simulink model "baseline_super_ground"  (R2021a)
settings: Solver=FixedStepAuto  StartTime=0.0  StopTime=50  FixedStep=framePeriod_s  RelTol=1e-3
undefined symbols (not defined in the file or in its folder): Aircraft, DiscIntNeverNeededParam, framePeriod_s
libraries: simulink x36
(part 1 of 2)
settings Model: Creator=brian  LastModifiedBy=Tuan Luong
settings SolverCC: AlgebraicLoopSolver=TrustRegion
settings OptimizationCC: DefaultParameterBehavior=Inlined  GainParamInheritBuiltInType=on  UseFloatMulNetSlope=on  DefaultUnderspecifiedDataType=single  InlineInvariantSignals=on  OptimizeBlockIOStorage=off  PassReuseOutputArgsAs=Individual arguments  ZeroExternalMemoryAtStartup=off  ZeroInternalMemoryAtStartup=off  NoFixptDivByZeroProtection=on  EfficientFloat2IntCast=on  LifeSpan=1  OptimizeBlockOrder=speed  DifferentSizesBufferReuse=on  EfficientTunableParamExpr=on
settings DebuggingCC: ParameterTunabilityLossMsg=error  SFMachineParentedDataDiag=warning
settings HardwareCC: ProdBitPerPointer=32  ProdBitPerSizeT=32  ProdBitPerPtrDiffT=32  ProdLargestAtomicInteger=Long  ProdLargestAtomicFloat=Double  ProdWordSize=32  ProdLongLongMode=on  ProdHWDeviceType=NXP->Cortex-M4
settings ModelReferenceCC: ModelReferenceNumInstancesAllowed=Single
settings SFSimCC: SimParseCustomCode=off  MATLABDynamicMemAlloc=off
settings RTWCC: SystemTargetFile=ert.tlc  GenCodeOnly=on  TemplateMakefile=ert_default_tmf  GenerateReport=on  RTWVerbose=off  Toolchain=Microsoft Visual C++ 2019 v16.0 | nmake (64-bit Windows)  BuildConfiguration=Faster Runs  IncludeHyperlinkInReport=on  TargetLang=C++  GenerateTraceInfo=on
settings CodeAppCC: ForceParamTrailComments=on  IgnoreCustomStorageClasses=off  OperatorAnnotations=on  SimulinkDataObjDesc=on  SFDataObjDesc=on  CustomSymbolStrGlobalVar=rt$N$M  CustomSymbolStrType=$N$M  CustomSymbolStrFcn=$N$M$F  CustomSymbolStrMacro=$N$M  InsertBlockDesc=on
settings ERTTargetCC: TargetLangStandard=C++03 (ISO)  IncludeMdlTerminateFcn=off  CombineSignalStateStructs=on  SuppressErrorStatus=on  SupportAbsoluteTime=off  CodeInterfacePackaging=C++ class  SupportComplex=off  ERTHeaderFileRootName=autocode$E  ERTSourceFileRootName=autocode$E  InlinedParameterPlacement=NonHierarchical  RootIOFormat=Structure reference  ERTCustomFileTemplate=example_file_process.tlc  ERTFilePackagingFormat=Compact  ArrayContainerType=std::array

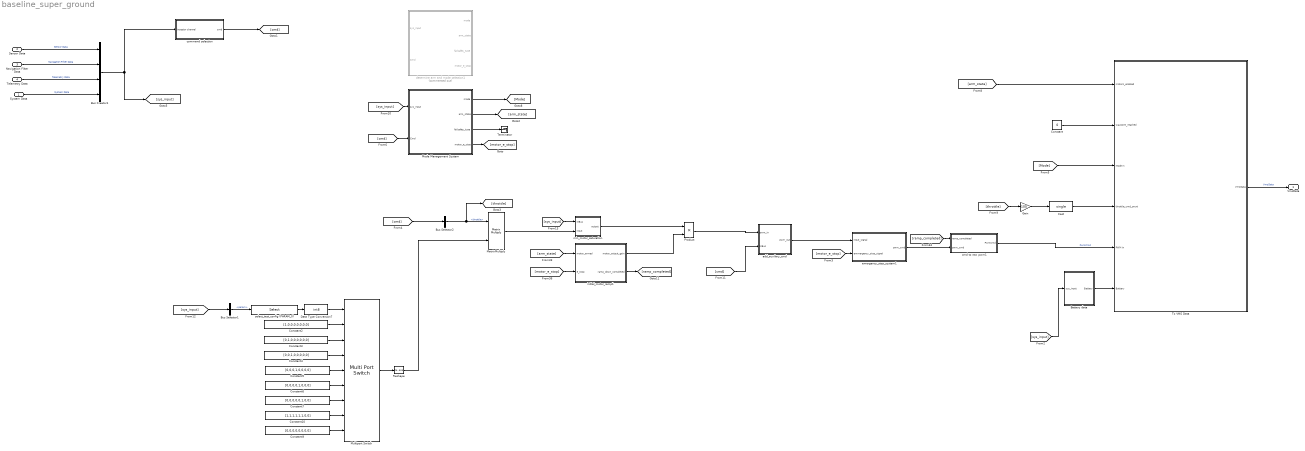
== system baseline_super_ground ==
  System Data : Inport  OutDataTypeStr=Bus: SysData  SampleTime=framePeriod_s  BusOutputAsStruct=on
  Sensor Data : Inport  Port=2  OutDataTypeStr=Bus: SensorData  SampleTime=framePeriod_s  BusOutputAsStruct=on
  Navigation Filter Data : Inport  Port=3  OutDataTypeStr=Bus: NavData  SampleTime=framePeriod_s  BusOutputAsStruct=on
  Telemetry Data : Inport  Port=4  OutDataTypeStr=Bus: TelemData  SampleTime=framePeriod_s  BusOutputAsStruct=on
  Battery data : Subsystem
  Bus Creator1 : BusCreator  Inputs=4
  Bus Selector1 : BusSelector  OutputSignals=Telemetry Data.param
  Bus Selector2 : BusSelector  OutputSignals=throttle
  Cast : DataTypeConversion  OutDataTypeStr=single
  Constant : Constant  Value=0  OutDataTypeStr=boolean
  Constant10 : Constant  Value=[1,1,1,1,1,1,0,0]  OutDataTypeStr=single
  Constant2 : Constant  Value=[1,0,0,0,0,0,0,0]  OutDataTypeStr=single
  Constant3 : Constant  Value=[0,1,0,0,0,0,0,0]  OutDataTypeStr=single
  Constant4 : Constant  Value=[0,0,1,0,0,0,0,0]  OutDataTypeStr=single
  Constant5 : Constant  Value=[0,0,0,1,0,0,0,0]  OutDataTypeStr=single
  Constant6 : Constant  Value=[0,0,0,0,1,0,0,0]  OutDataTypeStr=single
  Constant7 : Constant  Value=[0,0,0,0,0,1,0,0]  OutDataTypeStr=single
  Constant9 : Constant  Value=[0,0,0,0,0,0,0,0]  OutDataTypeStr=single
  Data Type Conversion7 : DataTypeConversion  OutDataTypeStr=int8
  Gain : Gain  Gain=100
  MatrixMultiply : Product  Multiplication=Matrix(*)
  Mode Management System : Subsystem
  Multiport Switch : MultiPortSwitch  DataPortOrder=Specify indices  Inputs=8  DataPortIndices={1,2,3,4,5,6,7}  DataPortForDefault=Additional data port
  Product : Product
  Reshape : Reshape  OutputDimensionality=Row vector (2-D)
  Terminator : Terminator
  To VMS Data : Subsystem
  add_auxilary_cmd : Subsystem
  cmd to raw pwm1 : Subsystem
  command selection : Subsystem
  determine arm and mode selection1 : Subsystem  Commented=on
  emergency_stop_system1 : Subsystem
  initial_motor_ramp1 : Subsystem
  min_motor_saturation : Subsystem
  select_test_config (PARAM_0) : Selector  IndexMode=Zero-based  IndexOptions=Index vector (dialog)  Indices=0  OutputSizes=1
  VmsData : Outport  OutDataTypeStr=Bus: VmsData  SampleTime=framePeriod_s  BusOutputAsStruct=on
  wires:
  Telemetry Data/1 -> Bus Creator1/3  "Telemetry Data"
  System Data/1 -> Bus Creator1/4  "System Data"
  Sensor Data/1 -> Bus Creator1/1  "Sensor Data"
  Navigation Filter Data/1 -> Bus Creator1/2  "Navigation Filter Data"
  To VMS Data/1(VmsData) -> VmsData/1  "VmsData"
  [Mode] -> To VMS Data/3(Mode in)
  Constant/1 -> To VMS Data/2(waypoint_reached)
  [arm_state] -> To VMS Data/1(motors_enabled)
  Cast/1 -> To VMS Data/4(throttle_cmd_prcnt)
  Battery data/1(Battery) -> To VMS Data/6(Battery)
  Bus Selector1/1 -> select_test_config (PARAM_0)/1  "<param>"
  select_test_config (PARAM_0)/1 -> Data Type Conversion7/1
  Data Type Conversion7/1 -> Multiport Switch/1
  [cmd] -> Bus Selector2/1
  Bus Selector2/1 -> [throttle], MatrixMultiply/1  "<throttle>"
  Multiport Switch/1 -> Reshape/1
  Reshape/1 -> MatrixMultiply/2
  [motor_e_stop] -> emergency_stop_system1/2(emmergency_stop_signal)
  initial_motor_ramp1/1(motor_output_gain) -> Product/2
  [sys_input] -> Battery data/1(sys_input)
  [throttle] -> Gain/1
  Gain/1 -> Cast/1
  Mode Management System/2(arm_state) -> [arm_state]
  command selection/1(cmd) -> [cmd]
  Mode Management System/3(failsafes_type) -> Terminator/1
  Mode Management System/1(mode) -> [Mode]
  Bus Creator1/1 -> command selection/1(inceptor channel), [sys_input]
  [cmd] -> Mode Management System/2(Cmd)
  [sys_input] -> Mode Management System/1(sys_input)
  Mode Management System/4(motor_e_stop) -> [motor_e_stop]
  Product/1 -> add_auxilary_cmd/1(pwm_in)
  add_auxilary_cmd/1(pwm_out) -> emergency_stop_system1/1(input_signal)
  [cmd] -> add_auxilary_cmd/2(InBus)
  Constant2/1 -> Multiport Switch/2
  Constant3/1 -> Multiport Switch/3
  Constant4/1 -> Multiport Switch/4
  Constant5/1 -> Multiport Switch/5
  Constant6/1 -> Multiport Switch/6
  Constant7/1 -> Multiport Switch/7
  Constant10/1 -> Multiport Switch/8
  Constant9/1 -> Multiport Switch/9
  [sys_input] -> Bus Selector1/1
  MatrixMultiply/1 -> min_motor_saturation/2(input)
  min_motor_saturation/1(output) -> Product/1
  [sys_input] -> min_motor_saturation/1(InBus)
  cmd to raw pwm1/1(PwmCmd) -> To VMS Data/5(PWM In)  "PwmCmd"
  emergency_stop_system1/1(pwm_cmd) -> cmd to raw pwm1/2(pwm_cmd)
  initial_motor_ramp1/2(ramp_down_completed) -> [ramp_completed]
  [arm_state] -> initial_motor_ramp1/1(motor_armed)
  [motor_e_stop] -> initial_motor_ramp1/2(e_stop)
  [ramp_completed] -> cmd to raw pwm1/1(ramp_completed)

== system baseline_super_ground/Battery data ==
  In Bus Element : Inport  PortName=sys_input  Element=Sensor Data.power_module.voltage_v
  In Bus Element1 : Inport  PortName=sys_input  Element=Sensor Data.power_module.current_v
  Bus Creator3 : BusCreator  Inputs=5  OutDataTypeStr=Bus: BatteryData  NonVirtualBus=on
  Discrete-Time Integrator : DiscreteIntegrator  IntegratorMethod=Integration: Trapezoidal  SampleTime=framePeriod_s  ICPrevOutput=DiscIntNeverNeededParam  ICPrevScaledInput=DiscIntNeverNeededParam
  Gain : Gain  Gain=Aircraft.Battery.voltage_gain
  Gain1 : Gain  Gain=Aircraft.Battery.current_to_voltage_gain_vpma
  remaining_prcnt : Constant  OutDataTypeStr=single
  remaining_time_s : Constant  OutDataTypeStr=single
  Battery : Outport
  wires:
  remaining_time_s/1 -> Bus Creator3/5  "remaining_time_s"
  Bus Creator3/1 -> Battery/1
  remaining_prcnt/1 -> Bus Creator3/4  "remaining_prcnt"
  In Bus Element1/1 -> Gain1/1
  Discrete-Time Integrator/1 -> Bus Creator3/3  "consumed_mah"
  In Bus Element/1 -> Gain/1
  Gain/1 -> Bus Creator3/1  "voltage_v"
  Gain1/1 -> Discrete-Time Integrator/1, Bus Creator3/2  "current_ma"

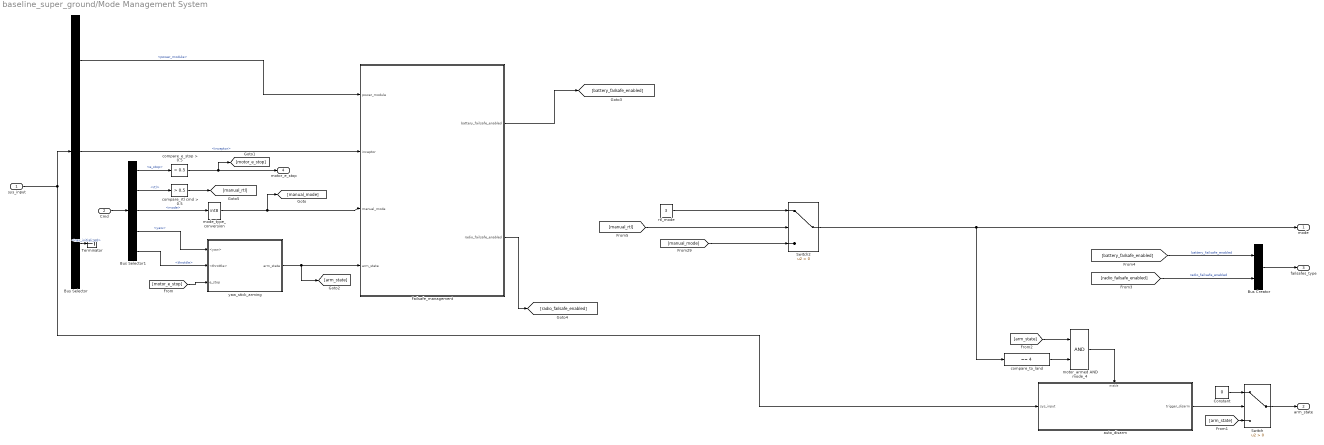
== system baseline_super_ground/Mode Management System ==
  sys_input : Inport
  Cmd : Inport  Port=2
  Bus Creator : BusCreator  Inputs=2
  Bus Selector : BusSelector  OutputSignals=Sensor Data.power_module,Sensor Data.inceptor,Navigation Filter Data.nav_initialized
  Bus Selector1 : BusSelector  OutputSignals=e_stop,rtl,mode,yaw,throttle
  Constant : Constant  Value=0  OutDataTypeStr=boolean
  Failsafe_management : Subsystem
  Switch : Switch  Criteria=u2 > Threshold
  Switch2 : Switch  Criteria=u2 > Threshold
  Terminator : Terminator
  auto_disarm : Subsystem
  compare_e_stop > 0.5 : simulink/Logic and Bit Operations/Compare To Constant  relop=>  const=0.5  OutDataTypeStr=boolean
  compare_rtl cmd > 0.5 : simulink/Logic and Bit Operations/Compare To Constant  relop=>  const=0.5  OutDataTypeStr=boolean
  compare_to_land : simulink/Logic and Bit Operations/Compare To Constant  relop===  const=4  OutDataTypeStr=boolean
  mode_type_conversion : DataTypeConversion  OutDataTypeStr=int8  RndMeth=Nearest
  motor_armed AND mode_4 : Logic  IconShape=distinctive  AllPortsSameDT=off  OutDataTypeStr=boolean
  rtl_mode : Constant  Value=3  OutDataTypeStr=int8
  yaw_stick_arming : Subsystem
  mode : Outport
  arm_state : Outport  Port=2
  failsafes_type : Outport  Port=3
  motor_e_stop : Outport  Port=4
  wires:
  mode_type_conversion/1 -> [manual_mode], Failsafe_management/3(manual_mode)
  rtl_mode/1 -> Switch2/1
  Failsafe_management/2(radio_failsafe_enabled) -> [radio_failsafe_enabled]
  [manual_mode] -> Switch2/3
  Failsafe_management/1(battery_failsafe_enabled) -> [battery_failsafe_enabled]
  Bus Selector/1 -> Failsafe_management/1(power_module)  "<power_module>"
  Bus Selector/2 -> Failsafe_management/2(inceptor)  "<inceptor>"
  sys_input/1 -> auto_disarm/1(sys_input), Bus Selector/1
  [arm_state] -> Switch/3
  auto_disarm/1(trigger_disarm) -> Switch/2
  Constant/1 -> Switch/1
  Switch/1 -> arm_state/1
  [arm_state] -> motor_armed AND mode_4/1
  compare_to_land/1 -> motor_armed AND mode_4/2
  Switch2/1 -> compare_to_land/1, mode/1
  motor_armed AND mode_4/1 -> auto_disarm/Enable
  [battery_failsafe_enabled] -> Bus Creator/1  "battery_failsafe_enabled"
  [radio_failsafe_enabled] -> Bus Creator/2  "radio_failsafe_enabled"
  Bus Creator/1 -> failsafes_type/1
  Cmd/1 -> Bus Selector1/1
  Bus Selector1/3 -> mode_type_conversion/1  "<mode>"
  Bus Selector1/2 -> compare_rtl cmd > 0.5/1  "<rtl>"
  compare_rtl cmd > 0.5/1 -> [manual_rtl]
  yaw_stick_arming/1(arm_state) -> Failsafe_management/4(arm_state), [arm_state]
  Bus Selector1/4 -> yaw_stick_arming/1(<yaw>)  "<yaw>"
  Bus Selector1/5 -> yaw_stick_arming/2(<throttle>)  "<throttle>"
  Bus Selector1/1 -> compare_e_stop > 0.5/1  "<e_stop>"
  compare_e_stop > 0.5/1 -> [motor_e_stop], motor_e_stop/1
  [manual_rtl] -> Switch2/2
  [motor_e_stop] -> yaw_stick_arming/3(e_stop)
  Bus Selector/3 -> Terminator/1  "<nav_initialized>"

== system baseline_super_ground/To VMS Data ==
  motors_enabled : Inport
  waypoint_reached : Inport  Port=2
  Mode in : Inport  Port=3
  throttle_cmd_prcnt : Inport  Port=4
  PWM In : Inport  Port=5
  Battery : Inport  Port=6
  Bus Creator : BusCreator  Inputs=9  OutDataTypeStr=Bus: VmsData  NonVirtualBus=on
  Bus Creator1 : BusCreator  Inputs=1  OutDataTypeStr=Bus: AnalogData
  Ground : Ground
  SBUS & AUX1 : Subsystem
  VmsData : Outport
  wires:
  waypoint_reached/1 -> Bus Creator/2  "waypoint_reached"
  Mode in/1 -> Bus Creator/3  "mode"
  motors_enabled/1 -> Bus Creator/1  "motors_enabled"
  Bus Creator/1 -> VmsData/1
  throttle_cmd_prcnt/1 -> Bus Creator/4  "throttle_cmd_prcnt"
  PWM In/1 -> Bus Creator/7  "pwm"
  SBUS & AUX1/1(aux) -> Bus Creator/5  "aux"
  SBUS & AUX1/2(sbus) -> Bus Creator/6  "SbusCmd"
  Battery/1 -> Bus Creator/9  "Battery"
  Bus Creator1/1 -> Bus Creator/8  "Analog"
  Ground/1 -> Bus Creator1/1  "val"

== system baseline_super_ground/add_auxilary_cmd ==
  pwm_in : Inport
  In Bus Element : Inport  Port=2  PortName=InBus  Element=engine
  In Bus Element1 : Inport  Port=2  PortName=InBus  Element=relay
  Demux : Demux  Outputs=8
  Mux : Mux  Inputs=8
  Sum : Sum  Inputs=|++
  Sum1 : Sum  Inputs=|++
  pwm_out : Outport
  wires:
  Demux/1 -> Mux/1  "motor1"
  Demux/2 -> Mux/2  "motor2"
  Demux/3 -> Mux/3  "motor3"
  Demux/6 -> Mux/6  "motor6"
  Demux/4 -> Mux/4  "motor4"
  Demux/5 -> Mux/5  "motor5"
  Mux/1 -> pwm_out/1
  pwm_in/1 -> Demux/1
  Demux/7 -> Sum/1
  Sum/1 -> Mux/7  "relay"
  Demux/8 -> Sum1/1
  Sum1/1 -> Mux/8  "engine"
  In Bus Element1/1 -> Sum/2
  In Bus Element/1 -> Sum1/2

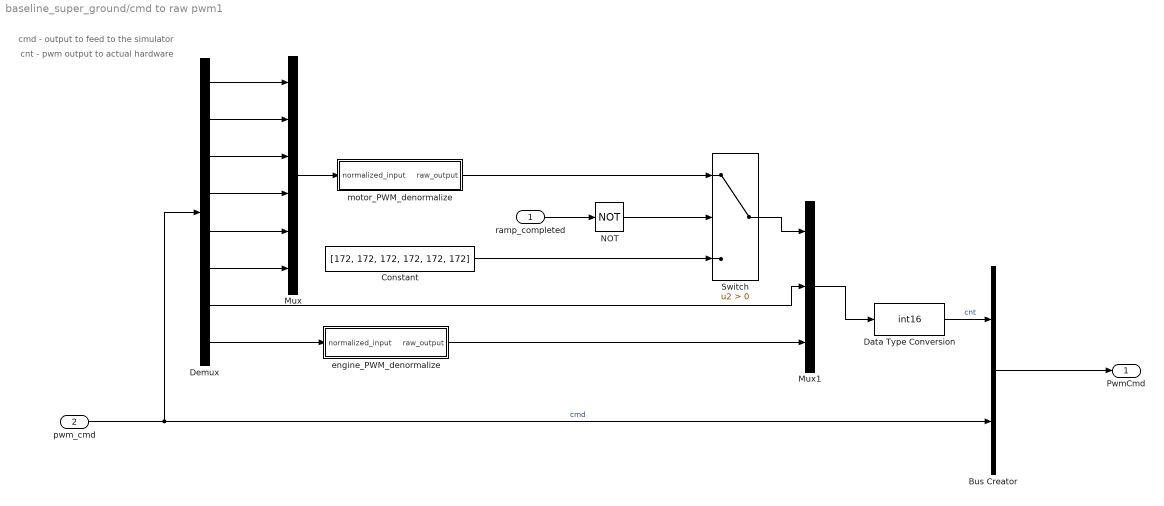
== system baseline_super_ground/cmd to raw pwm1 ==
  note: cnt - pwm output to actual hardware
  note: cmd - output to feed to the simulator
  ramp_completed : Inport
  pwm_cmd : Inport  Port=2
  Bus Creator : BusCreator  Inputs=2  OutDataTypeStr=Bus: PwmCmd  NonVirtualBus=on
      settings: InheritFromInputs=off
  Constant : Constant  Value=[172, 172, 172, 172, 172, 172]
  Data Type Conversion : DataTypeConversion  OutDataTypeStr=int16
  Demux : Demux  Outputs=8
  Mux : Mux  Inputs=6
  Mux1 : Mux  Inputs=3
  NOT : Logic  Operator=NOT  IconShape=distinctive  AllPortsSameDT=off  OutDataTypeStr=boolean
  Switch : Switch  Criteria=u2 > Threshold
  engine_PWM_denormalize : Subsystem
  motor_PWM_denormalize : Subsystem
  PwmCmd : Outport
  wires:
  Mux1/1 -> Data Type Conversion/1
  engine_PWM_denormalize/1(raw_output) -> Mux1/3
  Demux/7 -> Mux1/2
  Switch/1 -> Mux1/1
  Demux/8 -> engine_PWM_denormalize/1(normalized_input)
  motor_PWM_denormalize/1(raw_output) -> Switch/1
  Mux/1 -> motor_PWM_denormalize/1(normalized_input)
  Demux/6 -> Mux/6
  Demux/5 -> Mux/5
  Demux/4 -> Mux/4
  Demux/3 -> Mux/3
  Demux/2 -> Mux/2
  Demux/1 -> Mux/1
  Constant/1 -> Switch/3
  Data Type Conversion/1 -> Bus Creator/1  "cnt"
  pwm_cmd/1 -> Bus Creator/2, Demux/1  "cmd"
  Bus Creator/1 -> PwmCmd/1
  ramp_completed/1 -> NOT/1
  NOT/1 -> Switch/2

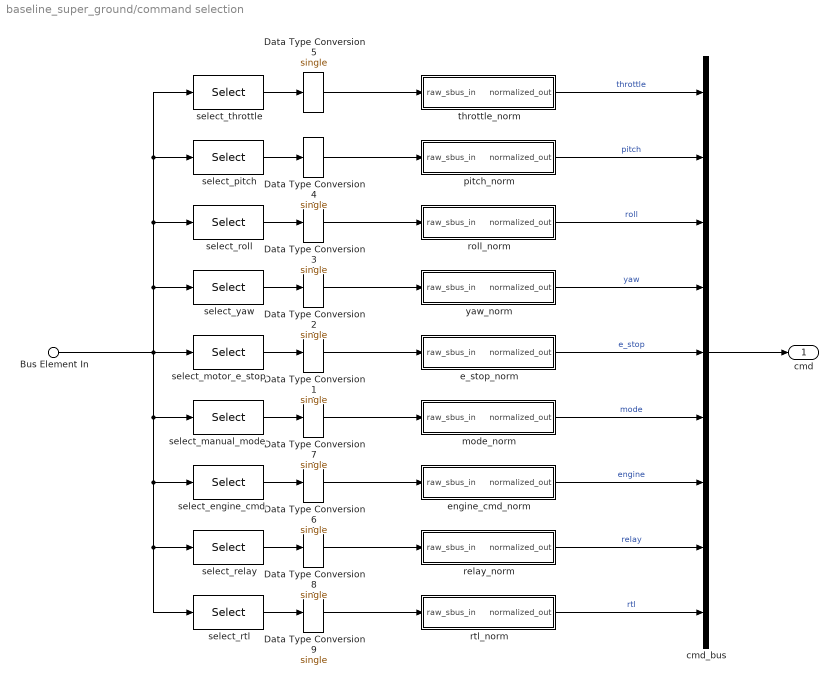
== system baseline_super_ground/command selection ==
  Bus Element In : Inport  PortName=inceptor channel  Element=Sensor Data.inceptor.ch
  Data Type Conversion{1..9} (9 alike) : DataTypeConversion  OutDataTypeStr=single
  cmd_bus : BusCreator  Inputs=9
  e_stop_norm : Subsystem
  engine_cmd_norm : Subsystem
  mode_norm : Subsystem
  pitch_norm : Subsystem
  relay_norm : Subsystem
  roll_norm : Subsystem
  rtl_norm : Subsystem
  select_engine_cmd : Selector  IndexOptions=Index vector (dialog)  Indices=Aircraft.Inceptor.engine_cmd  OutputSizes=1
  select_manual_mode : Selector  IndexOptions=Index vector (dialog)  Indices=Aircraft.Inceptor.mode0  OutputSizes=1
  select_motor_e_stop : Selector  IndexOptions=Index vector (dialog)  Indices=Aircraft.Inceptor.throttle_e_stop  OutputSizes=1
  select_pitch : Selector  IndexOptions=Index vector (dialog)  Indices=Aircraft.Inceptor.pitch  OutputSizes=1
  select_relay : Selector  IndexOptions=Index vector (dialog)  Indices=Aircraft.Inceptor.relay  OutputSizes=1
  select_roll : Selector  IndexOptions=Index vector (dialog)  Indices=Aircraft.Inceptor.roll  OutputSizes=1
  select_rtl : Selector  IndexOptions=Index vector (dialog)  Indices=Aircraft.Inceptor.rtl  OutputSizes=1
  select_throttle : Selector  IndexOptions=Index vector (dialog)  Indices=Aircraft.Inceptor.throttle  OutputSizes=1
  select_yaw : Selector  IndexOptions=Index vector (dialog)  Indices=Aircraft.Inceptor.yaw  OutputSizes=1
  throttle_norm : Subsystem
  yaw_norm : Subsystem
  cmd : Outport
  wires:
  select_pitch/1 -> Data Type Conversion4/1
  select_yaw/1 -> Data Type Conversion2/1
  Data Type Conversion2/1 -> yaw_norm/1(raw_sbus_in)
  select_throttle/1 -> Data Type Conversion5/1
  Data Type Conversion4/1 -> pitch_norm/1(raw_sbus_in)
  cmd_bus/1 -> cmd/1
  Data Type Conversion3/1 -> roll_norm/1(raw_sbus_in)
  Data Type Conversion5/1 -> throttle_norm/1(raw_sbus_in)
  select_roll/1 -> Data Type Conversion3/1
  Bus Element In/1 -> select_relay/1, select_rtl/1, select_engine_cmd/1, select_manual_mode/1, select_throttle/1, select_pitch/1, select_roll/1, select_yaw/1, select_motor_e_stop/1
  Data Type Conversion1/1 -> e_stop_norm/1(raw_sbus_in)
  select_motor_e_stop/1 -> Data Type Conversion1/1
  select_engine_cmd/1 -> Data Type Conversion6/1
  Data Type Conversion6/1 -> engine_cmd_norm/1(raw_sbus_in)
  Data Type Conversion7/1 -> mode_norm/1(raw_sbus_in)
  select_manual_mode/1 -> Data Type Conversion7/1
  select_relay/1 -> Data Type Conversion8/1
  Data Type Conversion8/1 -> relay_norm/1(raw_sbus_in)
  select_rtl/1 -> Data Type Conversion9/1
  Data Type Conversion9/1 -> rtl_norm/1(raw_sbus_in)
  throttle_norm/1(normalized_out) -> cmd_bus/1  "throttle"
  pitch_norm/1(normalized_out) -> cmd_bus/2  "pitch"
  roll_norm/1(normalized_out) -> cmd_bus/3  "roll"
  yaw_norm/1(normalized_out) -> cmd_bus/4  "yaw"
  e_stop_norm/1(normalized_out) -> cmd_bus/5  "e_stop"
  mode_norm/1(normalized_out) -> cmd_bus/6  "mode"
  engine_cmd_norm/1(normalized_out) -> cmd_bus/7  "engine"
  relay_norm/1(normalized_out) -> cmd_bus/8  "relay"
  rtl_norm/1(normalized_out) -> cmd_bus/9  "rtl"

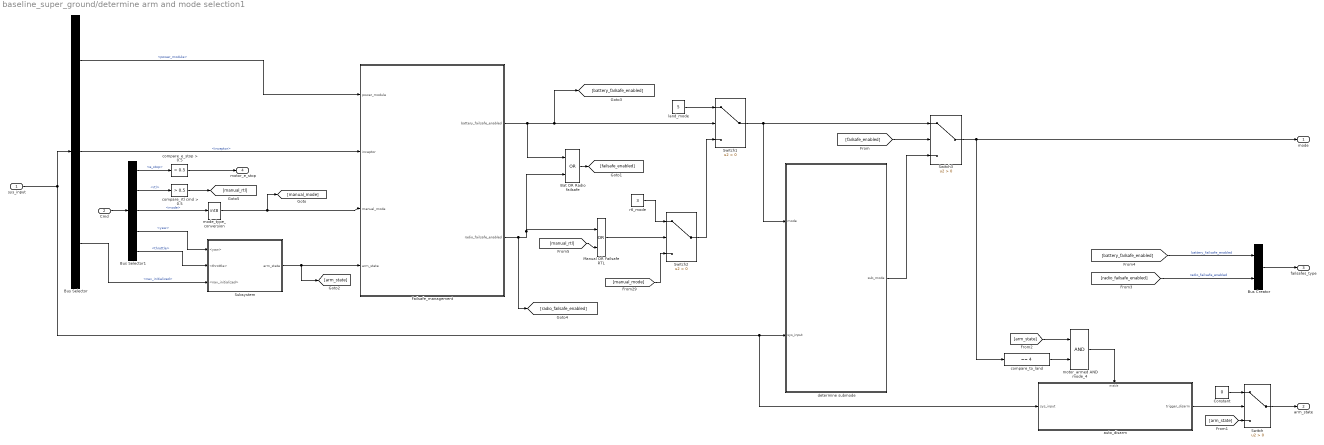
== system baseline_super_ground/determine arm and mode selection1 ==
  sys_input : Inport
  Cmd : Inport  Port=2
  Bat OR Radio failsafe : Logic  Operator=OR  IconShape=distinctive  AllPortsSameDT=off  OutDataTypeStr=boolean
  Bus Creator : BusCreator  Inputs=2
  Bus Selector : BusSelector  OutputSignals=Sensor Data.power_module,Sensor Data.inceptor,Navigation Filter Data.nav_initialized
  Bus Selector1 : BusSelector  OutputSignals=e_stop,rtl,mode,yaw,throttle
  Constant : Constant  Value=0  OutDataTypeStr=boolean
  Failsafe_management : Subsystem
  Manual OR Failsafe RTL : Logic  Operator=OR  IconShape=distinctive  AllPortsSameDT=off  OutDataTypeStr=boolean
  Subsystem : Subsystem
  Switch{,1..3} (4 alike) : Switch  Criteria=u2 > Threshold
  auto_disarm : Subsystem
  compare_e_stop > 0.5 : simulink/Logic and Bit Operations/Compare To Constant  relop=>  const=0.5  OutDataTypeStr=boolean
  compare_rtl cmd > 0.5 : simulink/Logic and Bit Operations/Compare To Constant  relop=>  const=0.5  OutDataTypeStr=boolean
  compare_to_land : simulink/Logic and Bit Operations/Compare To Constant  relop===  const=4  OutDataTypeStr=boolean
  determine submode : Subsystem
  land_mode : Constant  Value=5  OutDataTypeStr=int8
  mode_type_conversion : DataTypeConversion  OutDataTypeStr=int8  RndMeth=Nearest
  motor_armed AND mode_4 : Logic  IconShape=distinctive  AllPortsSameDT=off  OutDataTypeStr=boolean
  rtl_mode : Constant  Value=3  OutDataTypeStr=int8
  mode : Outport
  arm_state : Outport  Port=2
  failsafes_type : Outport  Port=3
  motor_e_stop : Outport  Port=4
  wires:
  mode_type_conversion/1 -> [manual_mode], Failsafe_management/3(manual_mode)
  rtl_mode/1 -> Switch2/1
  Failsafe_management/2(radio_failsafe_enabled) -> Bat OR Radio failsafe/2, Manual OR Failsafe RTL/1, [radio_failsafe_enabled]
  [manual_mode] -> Switch2/3
  land_mode/1 -> Switch1/1
  Failsafe_management/1(battery_failsafe_enabled) -> [battery_failsafe_enabled], Switch1/2, Bat OR Radio failsafe/1
  Bus Selector/3 -> Subsystem/3(<nav_initialized>)  "<nav_initialized>"
  Bus Selector/1 -> Failsafe_management/1(power_module)  "<power_module>"
  Bus Selector/2 -> Failsafe_management/2(inceptor)  "<inceptor>"
  Switch2/1 -> Switch1/3
  Bat OR Radio failsafe/1 -> [failsafe_enabled]
  sys_input/1 -> determine submode/2(sys_input), auto_disarm/1(sys_input), Bus Selector/1
  [failsafe_enabled] -> Switch3/2
  Switch1/1 -> Switch3/1, determine submode/1(mode)
  determine submode/1(sub_mode) -> Switch3/3
  [arm_state] -> Switch/3
  auto_disarm/1(trigger_disarm) -> Switch/2
  Constant/1 -> Switch/1
  Switch/1 -> arm_state/1
  [arm_state] -> motor_armed AND mode_4/1
  compare_to_land/1 -> motor_armed AND mode_4/2
  Switch3/1 -> compare_to_land/1, mode/1
  motor_armed AND mode_4/1 -> auto_disarm/Enable
  [battery_failsafe_enabled] -> Bus Creator/1  "battery_failsafe_enabled"
  [radio_failsafe_enabled] -> Bus Creator/2  "radio_failsafe_enabled"
  Bus Creator/1 -> failsafes_type/1
  Cmd/1 -> Bus Selector1/1
  Bus Selector1/3 -> mode_type_conversion/1  "<mode>"
  Manual OR Failsafe RTL/1 -> Switch2/2
  [manual_rtl] -> Manual OR Failsafe RTL/2
  Bus Selector1/2 -> compare_rtl cmd > 0.5/1  "<rtl>"
  compare_rtl cmd > 0.5/1 -> [manual_rtl]
  Subsystem/1(arm_state) -> Failsafe_management/4(arm_state), [arm_state]
  Bus Selector1/4 -> Subsystem/1(<yaw>)  "<yaw>"
  Bus Selector1/5 -> Subsystem/2(<throttle>)  "<throttle>"
  Bus Selector1/1 -> compare_e_stop > 0.5/1  "<e_stop>"
  compare_e_stop > 0.5/1 -> motor_e_stop/1

== system baseline_super_ground/emergency_stop_system1 ==
  input_signal : Inport
  emmergency_stop_signal : Inport  Port=2
  Constant : Constant  Value=[0,0,0,0,0,0,0,0]  OutDataTypeStr=single
  emergency_switch : Switch  Criteria=u2 > Threshold  Threshold=0.5
  pwm_cmd : Outport
  wires:
  emergency_switch/1 -> pwm_cmd/1
  emmergency_stop_signal/1 -> emergency_switch/2
  Constant/1 -> emergency_switch/1
  input_signal/1 -> emergency_switch/3

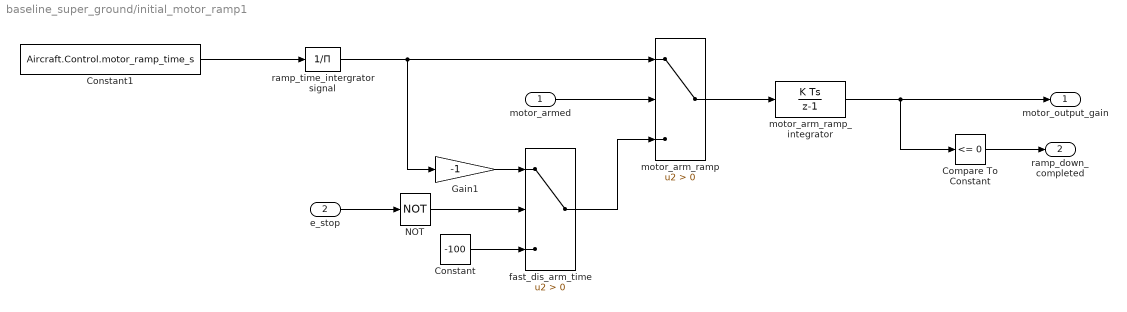
== system baseline_super_ground/initial_motor_ramp1 ==
  motor_armed : Inport
  e_stop : Inport  Port=2
  Compare To Constant : simulink/Logic and Bit Operations/Compare To Constant  relop=<=  const=0  OutDataTypeStr=boolean
  Constant : Constant  Value=-100
  Constant1 : Constant  Value=Aircraft.Control.motor_ramp_time_s  OutDataTypeStr=single
  Gain1 : Gain  Gain=-1
  NOT : Logic  Operator=NOT  IconShape=distinctive  AllPortsSameDT=off  OutDataTypeStr=boolean
  fast_dis_arm_time : Switch  Criteria=u2 > Threshold
  motor_arm_ramp : Switch  Criteria=u2 > Threshold
  motor_arm_ramp_integrator : DiscreteIntegrator  SampleTime=framePeriod_s  LimitOutput=on  UpperSaturationLimit=1  LowerSaturationLimit=0  ICPrevOutput=DiscIntNeverNeededParam  ICPrevScaledInput=DiscIntNeverNeededParam
  ramp_time_intergrator signal : Product  Inputs=/
  motor_output_gain : Outport
  ramp_down_completed : Outport  Port=2
  wires:
  Constant1/1 -> ramp_time_intergrator signal/1
  motor_arm_ramp/1 -> motor_arm_ramp_integrator/1
  ramp_time_intergrator signal/1 -> Gain1/1, motor_arm_ramp/1
  motor_arm_ramp_integrator/1 -> Compare To Constant/1, motor_output_gain/1
  motor_armed/1 -> motor_arm_ramp/2
  e_stop/1 -> NOT/1
  NOT/1 -> fast_dis_arm_time/2
  fast_dis_arm_time/1 -> motor_arm_ramp/3
  Gain1/1 -> fast_dis_arm_time/1
  Constant/1 -> fast_dis_arm_time/3
  Compare To Constant/1 -> ramp_down_completed/1

== system baseline_super_ground/min_motor_saturation ==
  In Bus Element : Inport  PortName=InBus  Element=Telemetry Data.param
  input : Inport  Port=2
  Constant : Constant
  Saturation Dynamic : simulink/Discontinuities/Saturation Dynamic  OutMin=[]  OutMax=[]  OutDataTypeStr=Inherit: Same as second input  OutDataType=fixdt(1, 16)  OutScaling=2^-10  DoSatur=off
  "min_motor_throttle (PARAM_1) " : Selector  IndexMode=Zero-based  IndexOptions=Index vector (dialog)  Indices=1  OutputSizes=1
  output : Outport
  wires:
  Constant/1 -> Saturation Dynamic/1
  input/1 -> Saturation Dynamic/2
  "min_motor_throttle (PARAM_1) "/1 -> Saturation Dynamic/3
  Saturation Dynamic/1 -> output/1
  In Bus Element/1 -> "min_motor_throttle (PARAM_1) "/1

== system baseline_super_ground/Mode Management System/Failsafe_management ==
  note: - radio failsafe
      | - battery failsafe
  Bus Element In : Inport  PortName=power_module  Element=voltage_v
  Bus Element In1 : Inport  Port=2  PortName=inceptor  Element=failsafe
  manual_mode : Inport  Port=3
  arm_state : Inport  Port=4
  Battery failsafe : Subsystem
  Radio failsafe : Subsystem
  battery_failsafe_enabled : Outport
  radio_failsafe_enabled : Outport  Port=2
  wires:
  Radio failsafe/1(radio_failsafe_enabled) -> radio_failsafe_enabled/1
  Battery failsafe/1(battery_failsafe_enabled) -> battery_failsafe_enabled/1
  manual_mode/1 -> [manual_mode], Radio failsafe/2(manual_mode)
  arm_state/1 -> Radio failsafe/3(arm_state), Battery failsafe/1(arm_state)
  [manual_mode] -> Battery failsafe/3(manual_mode)
  Bus Element In/1 -> Battery failsafe/2(voltage_v)
  Bus Element In1/1 -> Radio failsafe/1(failsafe)

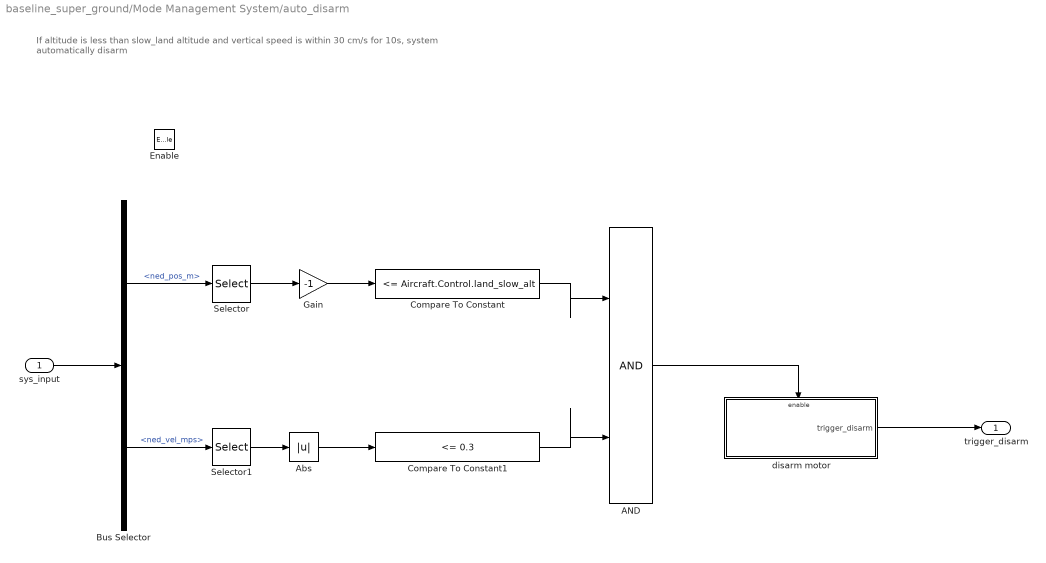
== system baseline_super_ground/Mode Management System/auto_disarm ==
  note: If altitude is less than slow_land altitude and vertical speed is within 30 cm/s for 10s, system automatically disarm
  sys_input : Inport
  Enable : EnablePort
  AND : Logic  IconShape=distinctive  AllPortsSameDT=off  OutDataTypeStr=boolean
  Abs : Abs
  Bus Selector : BusSelector  OutputSignals=Navigation Filter Data.ned_pos_m,Navigation Filter Data.ned_vel_mps
  Compare To Constant : simulink/Logic and Bit Operations/Compare To Constant  relop=<=  const=Aircraft.Control.land_slow_alt  OutDataTypeStr=boolean
  Compare To Constant1 : simulink/Logic and Bit Operations/Compare To Constant  relop=<=  const=0.3  OutDataTypeStr=boolean
  Gain : Gain  Gain=-1
  Selector : Selector  InputPortWidth=3  IndexOptions=Index vector (dialog)  Indices=3  OutputSizes=1
  Selector1 : Selector  InputPortWidth=3  IndexOptions=Index vector (dialog)  Indices=3  OutputSizes=1
  disarm motor : Subsystem
  trigger_disarm : Outport
  wires:
  sys_input/1 -> Bus Selector/1
  Bus Selector/1 -> Selector/1  "<ned_pos_m>"
  Bus Selector/2 -> Selector1/1  "<ned_vel_mps>"
  Selector/1 -> Gain/1
  Gain/1 -> Compare To Constant/1
  Selector1/1 -> Abs/1
  Abs/1 -> Compare To Constant1/1
  Compare To Constant/1 -> AND/1
  Compare To Constant1/1 -> AND/2
  AND/1 -> disarm motor/Enable
  disarm motor/1(trigger_disarm) -> trigger_disarm/1

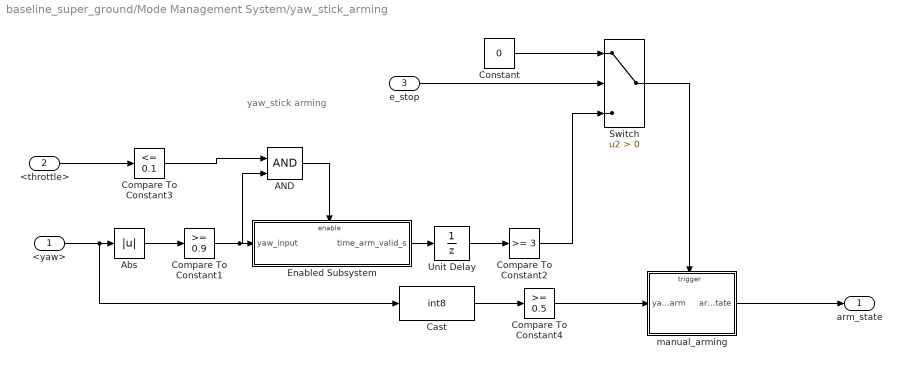
== system baseline_super_ground/Mode Management System/yaw_stick_arming ==
  note: yaw_stick arming
  <yaw> : Inport
  <throttle> : Inport  Port=2
  e_stop : Inport  Port=3
  AND : Logic  IconShape=distinctive  AllPortsSameDT=off  OutDataTypeStr=boolean
  Abs : Abs
  Cast : DataTypeConversion  OutDataTypeStr=int8
  Compare To Constant1 : simulink/Logic and Bit Operations/Compare To Constant  relop=>=  const=0.9  OutDataTypeStr=boolean
  Compare To Constant2 : simulink/Logic and Bit Operations/Compare To Constant  relop=>=  const=3  OutDataTypeStr=boolean
  Compare To Constant3 : simulink/Logic and Bit Operations/Compare To Constant  relop=<=  const=0.1  OutDataTypeStr=boolean
  Compare To Constant4 : simulink/Logic and Bit Operations/Compare To Constant  relop=>=  const=0.5  OutDataTypeStr=boolean
  Constant : Constant  Value=0  OutDataTypeStr=boolean  LockScale=on
  Enabled Subsystem : Subsystem  TreatAsAtomicUnit=on
  Switch : Switch  Criteria=u2 > Threshold
  Unit Delay : UnitDelay  SampleTime=-1  HasFrameUpgradeWarning=on
  manual_arming : Subsystem
  arm_state : Outport
  wires:
  Unit Delay/1 -> Compare To Constant2/1
  Abs/1 -> Compare To Constant1/1
  Enabled Subsystem/1(time_arm_valid_s) -> Unit Delay/1
  Compare To Constant1/1 -> AND/2, Enabled Subsystem/1(yaw_input)
  Compare To Constant4/1 -> manual_arming/1(yaw_arm)
  AND/1 -> Enabled Subsystem/Enable
  Cast/1 -> Compare To Constant4/1
  manual_arming/1(arm_state) -> arm_state/1
  <throttle>/1 -> Compare To Constant3/1
  <yaw>/1 -> Cast/1, Abs/1
  Switch/1 -> manual_arming/Trigger
  e_stop/1 -> Switch/2
  Constant/1 -> Switch/1
  Compare To Constant2/1 -> Switch/3
  Compare To Constant3/1 -> AND/1

== system baseline_super_ground/To VMS Data/SBUS & AUX1 ==
  Bus Creator : BusCreator  Inputs=4  OutDataTypeStr=Bus: SbusCmd  NonVirtualBus=on
  Constant : Constant  Value=0  OutDataTypeStr=boolean
  Constant1 : Constant  Value=0  OutDataTypeStr=boolean
  Data Type Conversion1 : DataTypeConversion  OutDataTypeStr=single
  Ground : Ground
  Ground1 : Ground
  Ground2 : Ground
  aux : Outport
  sbus : Outport  Port=2  SampleTime=framePeriod_s
  wires:
  Ground/1 -> Data Type Conversion1/1
  Data Type Conversion1/1 -> aux/1
  Bus Creator/1 -> sbus/1
  Constant/1 -> Bus Creator/1  "ch17"
  Constant1/1 -> Bus Creator/2  "ch18"
  Ground1/1 -> Bus Creator/3  "cnt"
  Ground2/1 -> Bus Creator/4  "cmd"

== system baseline_super_ground/cmd to raw pwm1/engine_PWM_denormalize ==
  normalized_input : Inport
  Constant : Constant  Value=0  OutDataTypeStr=single
  Constant1 : Constant  Value=900  OutDataTypeStr=single
  Constant2 : Constant  Value=2100  OutDataTypeStr=single
  Constant3 : Constant  OutDataTypeStr=single
  remap : MATLAB Function  TreatAsAtomicUnit=on
  raw_output : Outport
  wires:
  Constant2/1 -> remap/5(out_max)
  Constant1/1 -> remap/4(out_min)
  Constant3/1 -> remap/3(in_max)
  Constant/1 -> remap/2(in_min)
  remap/1(raw_out) -> raw_output/1
  normalized_input/1 -> remap/1(norm_in)

== system baseline_super_ground/cmd to raw pwm1/motor_PWM_denormalize ==
  normalized_input : Inport
  Constant : Constant  Value=0  OutDataTypeStr=single
  Constant1 : Constant  Value=1100  OutDataTypeStr=single
  Constant2 : Constant  Value=1900  OutDataTypeStr=single
  Constant3 : Constant  OutDataTypeStr=single
  remap : MATLAB Function  TreatAsAtomicUnit=on
  raw_output : Outport
  wires:
  Constant2/1 -> remap/5(out_max)
  Constant1/1 -> remap/4(out_min)
  Constant3/1 -> remap/3(in_max)
  Constant/1 -> remap/2(in_min)
  remap/1(raw_out) -> raw_output/1
  normalized_input/1 -> remap/1(norm_in)

== system baseline_super_ground/command selection/e_stop_norm ==
  raw_sbus_in : Inport
  Constant : Constant  Value=172  OutDataTypeStr=single
  Constant1 : Constant  Value=0  OutDataTypeStr=single
  Constant2 : Constant  OutDataTypeStr=single
  Constant3 : Constant  Value=1811  OutDataTypeStr=single
  remap : MATLAB Function  TreatAsAtomicUnit=on
  normalized_out : Outport
  wires:
  Constant2/1 -> remap/5(out_max)
  Constant1/1 -> remap/4(out_min)
  Constant3/1 -> remap/3(in_max)
  Constant/1 -> remap/2(in_min)
  remap/1(norm_out) -> normalized_out/1
  raw_sbus_in/1 -> remap/1(raw_in)

== system baseline_super_ground/command selection/engine_cmd_norm ==
  raw_sbus_in : Inport
  Constant : Constant  Value=172  OutDataTypeStr=single
  Constant1 : Constant  Value=0  OutDataTypeStr=single
  Constant2 : Constant  OutDataTypeStr=single
  Constant3 : Constant  Value=1811  OutDataTypeStr=single
  remap : MATLAB Function  TreatAsAtomicUnit=on
  normalized_out : Outport
  wires:
  Constant2/1 -> remap/5(out_max)
  Constant1/1 -> remap/4(out_min)
  Constant3/1 -> remap/3(in_max)
  Constant/1 -> remap/2(in_min)
  remap/1(norm_out) -> normalized_out/1
  raw_sbus_in/1 -> remap/1(raw_in)

== system baseline_super_ground/command selection/mode_norm ==
  raw_sbus_in : Inport
  Constant : Constant  Value=172  OutDataTypeStr=single
  Constant1 : Constant  Value=0  OutDataTypeStr=single
  Constant2 : Constant  Value=2  OutDataTypeStr=single
  Constant3 : Constant  Value=1811  OutDataTypeStr=single
  remap : MATLAB Function  TreatAsAtomicUnit=on
  normalized_out : Outport
  wires:
  raw_sbus_in/1 -> remap/1(raw_in)
  remap/1(norm_out) -> normalized_out/1
  Constant/1 -> remap/2(in_min)
  Constant3/1 -> remap/3(in_max)
  Constant1/1 -> remap/4(out_min)
  Constant2/1 -> remap/5(out_max)

== system baseline_super_ground/command selection/pitch_norm ==
  raw_sbus_in : Inport
  Constant : Constant  Value=172  OutDataTypeStr=single
  Constant1 : Constant  Value=-1  OutDataTypeStr=single
  Constant2 : Constant  OutDataTypeStr=single
  Constant3 : Constant  Value=1811  OutDataTypeStr=single
  remap : MATLAB Function  TreatAsAtomicUnit=on
  normalized_out : Outport
  wires:
  raw_sbus_in/1 -> remap/1(raw_in)
  remap/1(norm_out) -> normalized_out/1
  Constant/1 -> remap/2(in_min)
  Constant3/1 -> remap/3(in_max)
  Constant1/1 -> remap/4(out_min)
  Constant2/1 -> remap/5(out_max)

== system baseline_super_ground/command selection/relay_norm ==
  raw_sbus_in : Inport
  Constant : Constant  Value=172  OutDataTypeStr=single
  Constant1 : Constant  Value=0  OutDataTypeStr=single
  Constant2 : Constant  OutDataTypeStr=single
  Constant3 : Constant  Value=1811  OutDataTypeStr=single
  remap : MATLAB Function  TreatAsAtomicUnit=on
  normalized_out : Outport
  wires:
  raw_sbus_in/1 -> remap/1(raw_in)
  remap/1(norm_out) -> normalized_out/1
  Constant/1 -> remap/2(in_min)
  Constant3/1 -> remap/3(in_max)
  Constant1/1 -> remap/4(out_min)
  Constant2/1 -> remap/5(out_max)

== system baseline_super_ground/command selection/roll_norm ==
  raw_sbus_in : Inport
  Constant : Constant  Value=172  OutDataTypeStr=single
  Constant1 : Constant  Value=-1  OutDataTypeStr=single
  Constant2 : Constant  OutDataTypeStr=single
  Constant3 : Constant  Value=1811  OutDataTypeStr=single
  remap : MATLAB Function  TreatAsAtomicUnit=on
  normalized_out : Outport
  wires:
  Constant2/1 -> remap/5(out_max)
  Constant1/1 -> remap/4(out_min)
  Constant3/1 -> remap/3(in_max)
  Constant/1 -> remap/2(in_min)
  remap/1(norm_out) -> normalized_out/1
  raw_sbus_in/1 -> remap/1(raw_in)

== system baseline_super_ground/command selection/rtl_norm ==
  raw_sbus_in : Inport
  Constant : Constant  Value=172  OutDataTypeStr=single
  Constant1 : Constant  Value=0  OutDataTypeStr=single
  Constant2 : Constant  OutDataTypeStr=single
  Constant3 : Constant  Value=1811  OutDataTypeStr=single
  remap : MATLAB Function  TreatAsAtomicUnit=on
  normalized_out : Outport
  wires:
  Constant2/1 -> remap/5(out_max)
  Constant1/1 -> remap/4(out_min)
  Constant3/1 -> remap/3(in_max)
  Constant/1 -> remap/2(in_min)
  remap/1(norm_out) -> normalized_out/1
  raw_sbus_in/1 -> remap/1(raw_in)

== system baseline_super_ground/command selection/throttle_norm ==
  raw_sbus_in : Inport
  Constant : Constant  Value=172  OutDataTypeStr=single
  Constant1 : Constant  Value=0  OutDataTypeStr=single
  Constant2 : Constant  OutDataTypeStr=single
  Constant3 : Constant  Value=1811  OutDataTypeStr=single
  remap : MATLAB Function  TreatAsAtomicUnit=on
  normalized_out : Outport
  wires:
  raw_sbus_in/1 -> remap/1(raw_in)
  remap/1(norm_out) -> normalized_out/1
  Constant/1 -> remap/2(in_min)
  Constant3/1 -> remap/3(in_max)
  Constant1/1 -> remap/4(out_min)
  Constant2/1 -> remap/5(out_max)

== system baseline_super_ground/command selection/yaw_norm ==
  raw_sbus_in : Inport
  Constant : Constant  Value=172  OutDataTypeStr=single
  Constant1 : Constant  Value=-1  OutDataTypeStr=single
  Constant2 : Constant  OutDataTypeStr=single
  Constant3 : Constant  Value=1811  OutDataTypeStr=single
  remap : MATLAB Function  TreatAsAtomicUnit=on
  normalized_out : Outport
  wires:
  raw_sbus_in/1 -> remap/1(raw_in)
  remap/1(norm_out) -> normalized_out/1
  Constant/1 -> remap/2(in_min)
  Constant3/1 -> remap/3(in_max)
  Constant1/1 -> remap/4(out_min)
  Constant2/1 -> remap/5(out_max)

== system baseline_super_ground/determine arm and mode selection1/Failsafe_management ==
  note: - radio failsafe
      | - battery failsafe
  Bus Element In : Inport  PortName=power_module  Element=voltage_v
  Bus Element In1 : Inport  Port=2  PortName=inceptor  Element=failsafe
  manual_mode : Inport  Port=3
  arm_state : Inport  Port=4
  Battery failsafe : Subsystem
  Radio failsafe : Subsystem
  battery_failsafe_enabled : Outport
  radio_failsafe_enabled : Outport  Port=2
  wires:
  Radio failsafe/1(radio_failsafe_enabled) -> radio_failsafe_enabled/1
  Battery failsafe/1(battery_failsafe_enabled) -> battery_failsafe_enabled/1
  manual_mode/1 -> [manual_mode], Radio failsafe/2(manual_mode)
  arm_state/1 -> Radio failsafe/3(arm_state), Battery failsafe/1(arm_state)
  [manual_mode] -> Battery failsafe/3(manual_mode)
  Bus Element In/1 -> Battery failsafe/2(voltage_v)
  Bus Element In1/1 -> Radio failsafe/1(failsafe)

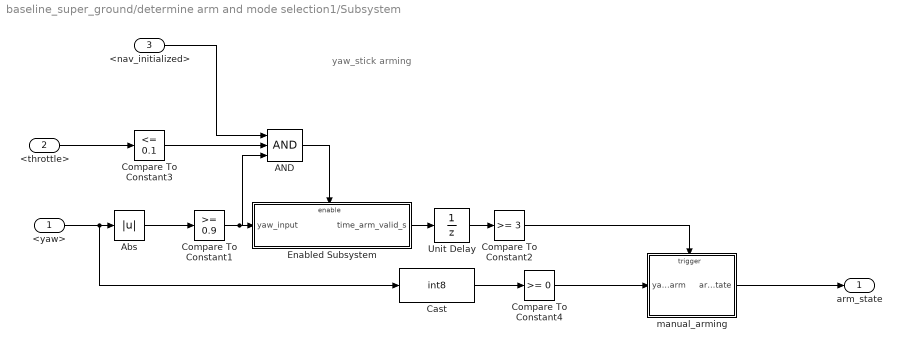
== system baseline_super_ground/determine arm and mode selection1/Subsystem ==
  note: yaw_stick arming
  <yaw> : Inport
  <throttle> : Inport  Port=2
  <nav_initialized> : Inport  Port=3
  AND : Logic  Inputs=3  IconShape=distinctive  AllPortsSameDT=off  OutDataTypeStr=boolean
  Abs : Abs
  Cast : DataTypeConversion  OutDataTypeStr=int8
  Compare To Constant1 : simulink/Logic and Bit Operations/Compare To Constant  relop=>=  const=0.9  OutDataTypeStr=boolean
  Compare To Constant2 : simulink/Logic and Bit Operations/Compare To Constant  relop=>=  const=3  OutDataTypeStr=boolean
  Compare To Constant3 : simulink/Logic and Bit Operations/Compare To Constant  relop=<=  const=0.1  OutDataTypeStr=boolean
  Compare To Constant4 : simulink/Logic and Bit Operations/Compare To Constant  relop=>=  const=0  OutDataTypeStr=boolean
  Enabled Subsystem : Subsystem  TreatAsAtomicUnit=on
  Unit Delay : UnitDelay  SampleTime=-1  HasFrameUpgradeWarning=on
  manual_arming : Subsystem
  arm_state : Outport
  wires:
  Unit Delay/1 -> Compare To Constant2/1
  Abs/1 -> Compare To Constant1/1
  Compare To Constant2/1 -> manual_arming/Trigger
  Enabled Subsystem/1(time_arm_valid_s) -> Unit Delay/1
  Compare To Constant1/1 -> AND/3, Enabled Subsystem/1(yaw_input)
  Compare To Constant4/1 -> manual_arming/1(yaw_arm)
  Compare To Constant3/1 -> AND/2
  AND/1 -> Enabled Subsystem/Enable
  Cast/1 -> Compare To Constant4/1
  manual_arming/1(arm_state) -> arm_state/1
  <throttle>/1 -> Compare To Constant3/1
  <nav_initialized>/1 -> AND/1
  <yaw>/1 -> Cast/1, Abs/1

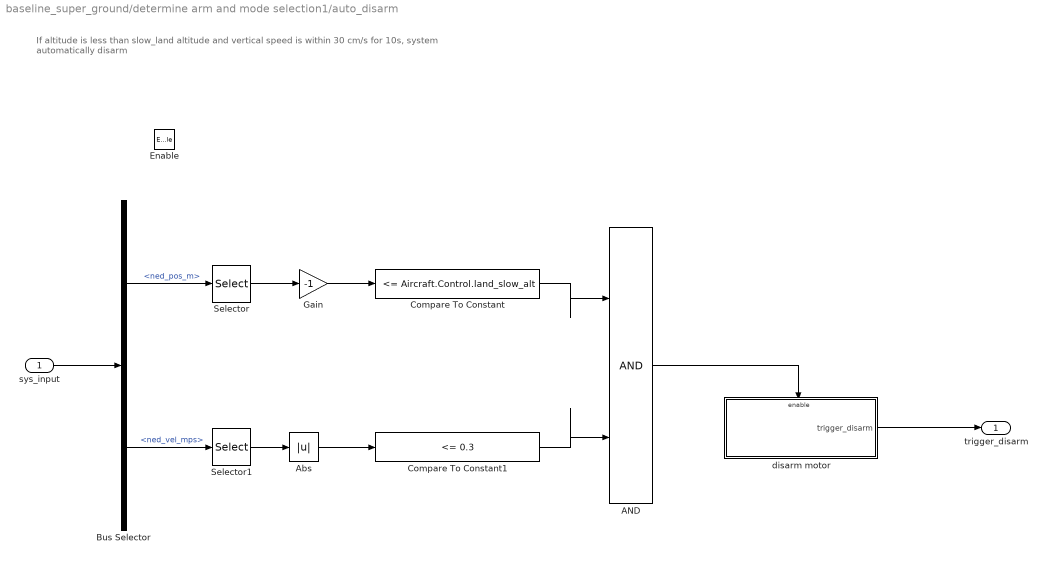
== system baseline_super_ground/determine arm and mode selection1/auto_disarm ==
  note: If altitude is less than slow_land altitude and vertical speed is within 30 cm/s for 10s, system automatically disarm
  sys_input : Inport
  Enable : EnablePort
  AND : Logic  IconShape=distinctive  AllPortsSameDT=off  OutDataTypeStr=boolean
  Abs : Abs
  Bus Selector : BusSelector  OutputSignals=Navigation Filter Data.ned_pos_m,Navigation Filter Data.ned_vel_mps
  Compare To Constant : simulink/Logic and Bit Operations/Compare To Constant  relop=<=  const=Aircraft.Control.land_slow_alt  OutDataTypeStr=boolean
  Compare To Constant1 : simulink/Logic and Bit Operations/Compare To Constant  relop=<=  const=0.3  OutDataTypeStr=boolean
  Gain : Gain  Gain=-1
  Selector : Selector  InputPortWidth=3  IndexOptions=Index vector (dialog)  Indices=3  OutputSizes=1
  Selector1 : Selector  InputPortWidth=3  IndexOptions=Index vector (dialog)  Indices=3  OutputSizes=1
  disarm motor : Subsystem
  trigger_disarm : Outport
  wires:
  sys_input/1 -> Bus Selector/1
  Bus Selector/1 -> Selector/1  "<ned_pos_m>"
  Bus Selector/2 -> Selector1/1  "<ned_vel_mps>"
  Selector/1 -> Gain/1
  Gain/1 -> Compare To Constant/1
  Selector1/1 -> Abs/1
  Abs/1 -> Compare To Constant1/1
  Compare To Constant/1 -> AND/1
  Compare To Constant1/1 -> AND/2
  AND/1 -> disarm motor/Enable
  disarm motor/1(trigger_disarm) -> trigger_disarm/1

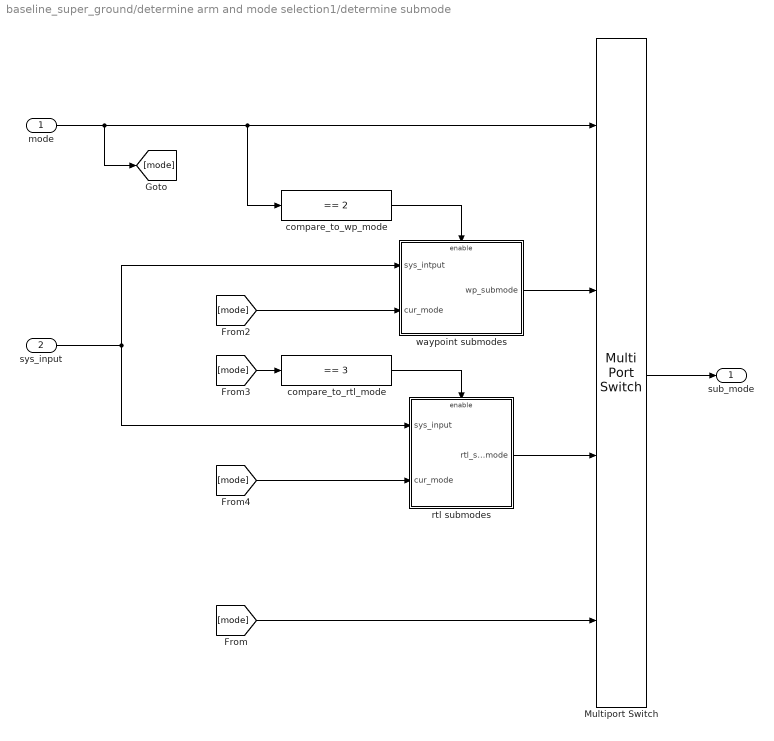
== system baseline_super_ground/determine arm and mode selection1/determine submode ==
  mode : Inport
  sys_input : Inport  Port=2
  Multiport Switch : MultiPortSwitch  DataPortOrder=Specify indices  DataPortIndices={2,3}  DataPortForDefault=Additional data port  DiagnosticForDefault=None
  compare_to_rtl_mode : simulink/Logic and Bit Operations/Compare To Constant  relop===  const=3  OutDataTypeStr=boolean
  compare_to_wp_mode : simulink/Logic and Bit Operations/Compare To Constant  relop===  const=2  OutDataTypeStr=boolean
  rtl submodes : Subsystem
  waypoint submodes : Subsystem
  sub_mode : Outport
  wires:
  compare_to_wp_mode/1 -> waypoint submodes/Enable
  waypoint submodes/1(wp_submode) -> Multiport Switch/2
  sys_input/1 -> rtl submodes/1(sys_input), waypoint submodes/1(sys_intput)
  Multiport Switch/1 -> sub_mode/1
  mode/1 -> [mode], compare_to_wp_mode/1, Multiport Switch/1
  [mode] -> waypoint submodes/2(cur_mode)
  [mode] -> compare_to_rtl_mode/1
  compare_to_rtl_mode/1 -> rtl submodes/Enable
  [mode] -> rtl submodes/2(cur_mode)
  rtl submodes/1(rtl_submode) -> Multiport Switch/3
  [mode] -> Multiport Switch/4

== system baseline_super_ground/Mode Management System/Failsafe_management/Battery failsafe ==
  note: Land immediatedly
  note: Battery voltage is less than 46.8 for more than 15 seconds and current_mode is not Land nor arm_state is off
  arm_state : Inport
  voltage_v : Inport  Port=2
  manual_mode : Inport  Port=3
  AND : Logic  Inputs=3  IconShape=distinctive  AllPortsSameDT=off  OutDataTypeStr=boolean
  Compare To Constant : simulink/Logic and Bit Operations/Compare To Constant  relop=~=  const=5  OutDataTypeStr=boolean
  Compare To Constant3 : simulink/Logic and Bit Operations/Compare To Constant  relop=<=  const=46.8  OutDataTypeStr=boolean
  disarm motor : Subsystem
  battery_failsafe_enabled : Outport
  wires:
  Compare To Constant/1 -> AND/2
  AND/1 -> battery_failsafe_enabled/1
  manual_mode/1 -> Compare To Constant/1
  Compare To Constant3/1 -> disarm motor/Enable
  disarm motor/1(battery_low_trigger) -> AND/1
  arm_state/1 -> AND/3
  voltage_v/1 -> Compare To Constant3/1

== system baseline_super_ground/Mode Management System/Failsafe_management/Radio failsafe ==
  note: Transition to RTL mode
  note: If radio_failsafe is triggered and current_mode is not auto, rtl, land nor motor_state disarmed then RTL mode is triggered
  failsafe : Inport
  manual_mode : Inport  Port=2
  arm_state : Inport  Port=3
  AND : Logic  IconShape=distinctive  AllPortsSameDT=off  OutDataTypeStr=boolean
  Compare To Constant : simulink/Logic and Bit Operations/Compare To Constant  relop=~=  const=3  OutDataTypeStr=boolean
  Compare To Constant1 : simulink/Logic and Bit Operations/Compare To Constant  relop=~=  const=4  OutDataTypeStr=boolean
  Compare To Constant2 : simulink/Logic and Bit Operations/Compare To Constant  relop=~=  const=5  OutDataTypeStr=boolean
  NOR : Logic  Operator=NOR  Inputs=4  IconShape=distinctive  AllPortsSameDT=off  OutDataTypeStr=boolean
  NOT : Logic  Operator=NOT  IconShape=distinctive  AllPortsSameDT=off  OutDataTypeStr=boolean
  radio_failsafe_enabled : Outport
  wires:
  NOR/1 -> AND/2
  manual_mode/1 -> Compare To Constant2/1, Compare To Constant1/1, Compare To Constant/1
  AND/1 -> radio_failsafe_enabled/1
  Compare To Constant/1 -> NOR/1
  Compare To Constant1/1 -> NOR/2
  Compare To Constant2/1 -> NOR/3
  arm_state/1 -> NOT/1
  NOT/1 -> NOR/4
  failsafe/1 -> AND/1

== system baseline_super_ground/Mode Management System/auto_disarm/disarm motor ==
  Enable : EnablePort  StatesWhenEnabling=reset
  Compare To Constant2 : simulink/Logic and Bit Operations/Compare To Constant  relop=>  const=10  OutDataTypeStr=boolean
  Constant : Constant  Value=framePeriod_s
  Sum : Sum  Inputs=|++
  Unit Delay : UnitDelay  SampleTime=-1  HasFrameUpgradeWarning=on
  trigger_disarm : Outport
  wires:
  Compare To Constant2/1 -> trigger_disarm/1
  Sum/1 -> Compare To Constant2/1, Unit Delay/1
  Unit Delay/1 -> Sum/2
  Constant/1 -> Sum/1

== system baseline_super_ground/Mode Management System/yaw_stick_arming/Enabled Subsystem ==
  yaw_input : Inport
  Enable : EnablePort  StatesWhenEnabling=reset
  Cast : DataTypeConversion  OutDataTypeStr=int8
  Discrete-Time Integrator : DiscreteIntegrator  IntegratorMethod=Integration: Trapezoidal  SampleTime=-1  OutDataTypeStr=single  UpperSaturationLimit=1  LowerSaturationLimit=0  ICPrevOutput=DiscIntNeverNeededParam  ICPrevScaledInput=DiscIntNeverNeededParam
  time_arm_valid_s : Outport
  wires:
  Discrete-Time Integrator/1 -> time_arm_valid_s/1
  Cast/1 -> Discrete-Time Integrator/1
  yaw_input/1 -> Cast/1

== system baseline_super_ground/Mode Management System/yaw_stick_arming/manual_arming ==
  yaw_arm : Inport
  Trigger : TriggerPort  TriggerType=either  VariantControl=(inherit)  PortDimensions=1
  arm_state : Outport
  wires:
  yaw_arm/1 -> arm_state/1

== system baseline_super_ground/determine arm and mode selection1/Failsafe_management/Battery failsafe ==
  note: Land immediatedly
  note: Battery voltage is less than 46.8 for more than 15 seconds and current_mode is not Land nor arm_state is off
  arm_state : Inport
  voltage_v : Inport  Port=2
  manual_mode : Inport  Port=3
  AND : Logic  Inputs=3  IconShape=distinctive  AllPortsSameDT=off  OutDataTypeStr=boolean
  Compare To Constant : simulink/Logic and Bit Operations/Compare To Constant  relop=~=  const=5  OutDataTypeStr=boolean
  Compare To Constant3 : simulink/Logic and Bit Operations/Compare To Constant  relop=<=  const=46.8  OutDataTypeStr=boolean
  disarm motor : Subsystem
  battery_failsafe_enabled : Outport
  wires:
  Compare To Constant/1 -> AND/2
  AND/1 -> battery_failsafe_enabled/1
  manual_mode/1 -> Compare To Constant/1
  Compare To Constant3/1 -> disarm motor/Enable
  disarm motor/1(battery_low_trigger) -> AND/1
  arm_state/1 -> AND/3
  voltage_v/1 -> Compare To Constant3/1

== system baseline_super_ground/determine arm and mode selection1/Failsafe_management/Radio failsafe ==
  note: Transition to RTL mode
  note: If radio_failsafe is triggered and current_mode is not auto, rtl, land nor motor_state disarmed then RTL mode is triggered
  failsafe : Inport
  manual_mode : Inport  Port=2
  arm_state : Inport  Port=3
  AND : Logic  IconShape=distinctive  AllPortsSameDT=off  OutDataTypeStr=boolean
  Compare To Constant : simulink/Logic and Bit Operations/Compare To Constant  relop=~=  const=3  OutDataTypeStr=boolean
  Compare To Constant1 : simulink/Logic and Bit Operations/Compare To Constant  relop=~=  const=4  OutDataTypeStr=boolean
  Compare To Constant2 : simulink/Logic and Bit Operations/Compare To Constant  relop=~=  const=5  OutDataTypeStr=boolean
  NOR : Logic  Operator=NOR  Inputs=4  IconShape=distinctive  AllPortsSameDT=off  OutDataTypeStr=boolean
  NOT : Logic  Operator=NOT  IconShape=distinctive  AllPortsSameDT=off  OutDataTypeStr=boolean
  radio_failsafe_enabled : Outport
  wires:
  NOR/1 -> AND/2
  manual_mode/1 -> Compare To Constant2/1, Compare To Constant1/1, Compare To Constant/1
  AND/1 -> radio_failsafe_enabled/1
  Compare To Constant/1 -> NOR/1
  Compare To Constant1/1 -> NOR/2
  Compare To Constant2/1 -> NOR/3
  arm_state/1 -> NOT/1
  NOT/1 -> NOR/4
  failsafe/1 -> AND/1

== system baseline_super_ground/determine arm and mode selection1/Subsystem/Enabled Subsystem ==
  yaw_input : Inport
  Enable : EnablePort  StatesWhenEnabling=reset
  Cast : DataTypeConversion  OutDataTypeStr=int8
  Discrete-Time Integrator : DiscreteIntegrator  IntegratorMethod=Integration: Trapezoidal  SampleTime=-1  OutDataTypeStr=single  UpperSaturationLimit=1  LowerSaturationLimit=0  ICPrevOutput=DiscIntNeverNeededParam  ICPrevScaledInput=DiscIntNeverNeededParam
  time_arm_valid_s : Outport
  wires:
  Discrete-Time Integrator/1 -> time_arm_valid_s/1
  Cast/1 -> Discrete-Time Integrator/1
  yaw_input/1 -> Cast/1

== system baseline_super_ground/determine arm and mode selection1/Subsystem/manual_arming ==
  yaw_arm : Inport
  Trigger : TriggerPort  VariantControl=(inherit)  PortDimensions=1
  arm_state : Outport
  wires:
  yaw_arm/1 -> arm_state/1

== system baseline_super_ground/determine arm and mode selection1/auto_disarm/disarm motor ==
  Enable : EnablePort  StatesWhenEnabling=reset
  Compare To Constant2 : simulink/Logic and Bit Operations/Compare To Constant  relop=>  const=10  OutDataTypeStr=boolean
  Constant : Constant  Value=framePeriod_s
  Sum : Sum  Inputs=|++
  Unit Delay : UnitDelay  SampleTime=-1  HasFrameUpgradeWarning=on
  trigger_disarm : Outport
  wires:
  Compare To Constant2/1 -> trigger_disarm/1
  Sum/1 -> Compare To Constant2/1, Unit Delay/1
  Unit Delay/1 -> Sum/2
  Constant/1 -> Sum/1

== system baseline_super_ground/determine arm and mode selection1/determine submode/rtl submodes ==
  note: Fast RTL check if UAV already within WP radius of the home position so that it can Land right away
  sys_input : Inport
  cur_mode : Inport  Port=2
  Enable : EnablePort
  Bus Selector : BusSelector  OutputSignals=Navigation Filter Data.ned_pos_m
  Constant : Constant  Value=Aircraft.Control.wp_radius
  Constant1 : Constant  Value=[0,0,0]  OutDataTypeStr=single
  determine_fast_rtl_mode : MATLAB Function  TreatAsAtomicUnit=on
  rtl_submode : Outport
  wires:
  Constant1/1 -> determine_fast_rtl_mode/1(target_pos)
  sys_input/1 -> Bus Selector/1
  Bus Selector/1 -> determine_fast_rtl_mode/2(ned_pos)  "<ned_pos_m>"
  determine_fast_rtl_mode/1(sub_mode) -> rtl_submode/1
  cur_mode/1 -> determine_fast_rtl_mode/3(cur_mode)
  Constant/1 -> determine_fast_rtl_mode/4(Aircraft_Control_wp_radius)
